simulink model "prueba"  (R2021a)
settings: Solver=FixedStepAuto  StartTime=0.0  StopTime=inf  FixedStep=0.001  MaxStep=1e-4  RelTol=1e-3
settings Model: SimulationMode=accelerator  Creator=Mariano  LastModifiedBy=facu_
settings SolverCC: ODENIntegrationMethod=ode2

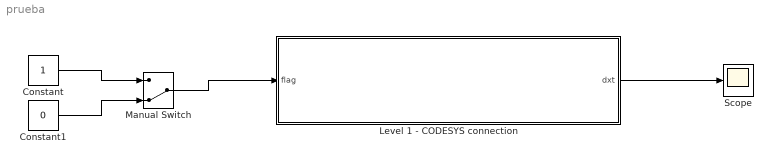
== system prueba ==
  Constant : Constant
  Constant1 : Constant  Value=0
  Level 1 - CODESYS connection : Subsystem  TreatAsAtomicUnit=on  SystemSampleTime=0.1
  Manual Switch : ManualSwitch  CurrentSetting=0
  Scope : Scope
  wires:
  Manual Switch/1 -> Level 1 - CODESYS connection/1(flag)
  Constant/1 -> Manual Switch/1
  Constant1/1 -> Manual Switch/2
  Level 1 - CODESYS connection/1(dxt) -> Scope/1

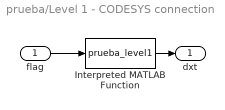
== system prueba/Level 1 - CODESYS connection ==
  flag : Inport
  Interpreted MATLAB Function : MATLABFcn  MATLABFcn=prueba_level1
  dxt : Outport
  wires:
  flag/1 -> Interpreted MATLAB Function/1
  Interpreted MATLAB Function/1 -> dxt/1
